simulink model "Planta_Matlab"  (R2017a)
settings: Solver=VariableStepAuto  StartTime=0.0  StopTime=0.4  MaxStep=1e-4  RelTol=1e-3
libraries: powerlib x20, opclib x10, simulink x7, powerlib_meascontrol x3, re_lib x1
settings Model: Creator=lideq2  LastModifiedBy=igor-
settings SolverCC: MaxConsecutiveZCs=10000

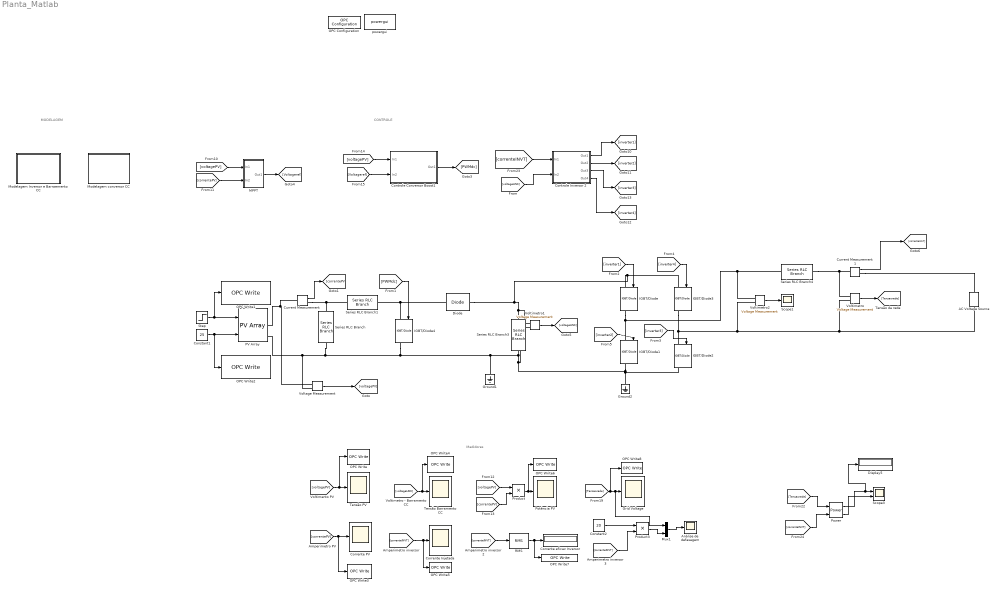
== system Planta_Matlab ==
  note: CONTROLE
  note: Medidores
  note: MODELAGEM
  AC Voltage Source : powerlib/Electrical Sources/AC Voltage Source  Amplitude=325  Phase=0  Frequency=60  SampleTime=0  Measurements=None  BusType=swing  Pref=10e3  Qref=0  Qmin=-inf  Qmax=+inf
  Análise de defasagem : Scope
  Constant1 : Constant  Value=25
  Constant2 : Constant  Value=20
  Controle Conversor Boost1 : Subsystem
  Controle Inversor 2 : Subsystem
  Corrente Injetada : Scope
  "Corrente PV " : Scope
  Corrente eficaz Inversor : Display
  Current Measurement : powerlib/Measurements/Current Measurement  PhasorSimulation=off  OutputType=Complex  PSBequivalent=0
  Current Measurement1 : powerlib/Measurements/Current Measurement  PhasorSimulation=off  OutputType=Complex  PSBequivalent=0
  Diode : powerlib/Power Electronics/Diode  Ron=0.001  Lon=0  Vf=0.8  IC=0  UseSnubber=off  Rs=500  Cs=250e-9  Measurements=off
  Display5 : Display
  Grid Voltage : Scope
  Ground1 : powerlib/Elements/Ground  LConnTagsString=a
  Ground2 : powerlib/Elements/Ground  LConnTagsString=a
  IGBT/Diode{,1..4} (5 alike) : powerlib/Power Electronics/IGBT//Diode  Ron=1e-3  Rs=1e5  Cs=inf  Measurements=on
  MPPT : Subsystem
  Modelagem Inversor e Barraemento CC : Subsystem
  Modelagem conversor CC : Subsystem
  Mux1 : Mux  Inputs=2
  OPC Configuration : opclib/OPC Configuration  opcServers=localhost/Matrikon.OPC.Simulation.1/10  errMissingItems=Error  errReadWrite=Warn  errShutdown=Error  errRTViolation=Warn  rtEnable=on  speedup=1  showLatency=off  beingUsed=on
      settings: SourceProductName=OPC Toolbox  SourceProductBaseCode=OT
  OPC Write : opclib/OPC Write  serverHost=localhost  serverID=Matrikon.OPC.Simulation.1  itemIDs=PV_v2.Placa.Tensão_PV  writeMode=Synchronous  updateRate=0
      settings: SourceProductName=OPC Toolbox  SourceProductBaseCode=OT
  OPC Write1 : opclib/OPC Write  serverHost=localhost  serverID=Matrikon.OPC.Simulation.1  itemIDs=PV_v2.Placa.IRRADIANCIA  writeMode=Synchronous  updateRate=0
      settings: SourceProductName=OPC Toolbox  SourceProductBaseCode=OT
  OPC Write2 : opclib/OPC Write  serverHost=localhost  serverID=Matrikon.OPC.Simulation.1  itemIDs=PV_v2.Placa.TEMPERATURA  writeMode=Synchronous  updateRate=0
      settings: SourceProductName=OPC Toolbox  SourceProductBaseCode=OT
  OPC Write3 : opclib/OPC Write  serverHost=localhost  serverID=Matrikon.OPC.Simulation.1  itemIDs=PV_v2.Placa.Corrente_PV  writeMode=Synchronous  updateRate=0
      settings: SourceProductName=OPC Toolbox  SourceProductBaseCode=OT
  OPC Write4 : opclib/OPC Write  serverHost=localhost  serverID=Matrikon.OPC.Simulation.1  itemIDs=PV_v2.Placa.Tensão_Barramento  writeMode=Synchronous  updateRate=0
      settings: SourceProductName=OPC Toolbox  SourceProductBaseCode=OT
  OPC Write5 : opclib/OPC Write  serverHost=localhost  serverID=Matrikon.OPC.Simulation.1  itemIDs=PV_v2.Inversor.Corrente_Injetada  writeMode=Synchronous  updateRate=0
      settings: SourceProductName=OPC Toolbox  SourceProductBaseCode=OT
  OPC Write6 : opclib/OPC Write  serverHost=localhost  serverID=Matrikon.OPC.Simulation.1  itemIDs=PV_v2.Placa.Potência_PV  writeMode=Synchronous  updateRate=0
      settings: SourceProductName=OPC Toolbox  SourceProductBaseCode=OT
  OPC Write7 : opclib/OPC Write  serverHost=localhost  serverID=Matrikon.OPC.Simulation.1  itemIDs=PV_v2.Inversor.Corrente_Eficaz_INV  writeMode=Synchronous  updateRate=0
      settings: SourceProductName=OPC Toolbox  SourceProductBaseCode=OT
  OPC Write8 : opclib/OPC Write  serverHost=localhost  serverID=Matrikon.OPC.Simulation.1  itemIDs=PV_v2.Rede.Tensão_Rede  writeMode=Synchronous  updateRate=0
      settings: SourceProductName=OPC Toolbox  SourceProductBaseCode=OT
  PV Array : re_lib/Solar/PV Array  Npar=1  Nser=5  PlotType=array @ 1000 W/m2 & specified temperatures  S_vec="[ 1000  500  100 ]"  Temp_C_vec="[ 45 25  ]"  ModuleName=Yingli Energy (China) YL240P-29b  PlotWhenSelected=off  Pm=240.13  Ncell=60  Voc=37.5  Isc=8.65  Vm=29.5  Im=8.14  beta_Voc_pc=-0.33701  alpha_Isc_pc=0.043803  beta_Voc=-0.12638  alpha_Isc=0.003789  IL=8.6929  I0=1.2567e-10  nI=0.97513  Rsh=337.0126  Rs=0.44582  BAL=off  Tc=1e-6  Tfilter=5e-5
  Potência PV : Scope
  Power : powerlib_meascontrol/Measurements/Power  Freq=60  Vinit=[1, 0]  Iinit=[1, 0]  Ts=1e-6
      settings: SourceProductName=Simscape Power Systems
  Product : Product
  Product3 : Product
  RMS : powerlib_meascontrol/Measurements/RMS  TrueRMS=on  Freq=60  RMSInit=120  Ts=0
  Scope1 : Scope
  Scope3 : Scope  NumInputPorts=2
  Series RLC Branch : powerlib/Elements/Series RLC Branch  LConnTagsString=__new0  RConnTagsString=__new0  BranchType=C  Resistance=1  Inductance=1e-3  SetiL0=off  InitialCurrent=0  Capacitance=1e-3  Setx0=off  InitialVoltage=0  Measurements=None
  Series RLC Branch1 : powerlib/Elements/Series RLC Branch  LConnTagsString=__new0  RConnTagsString=__new0  BranchType=L  Resistance=1  Inductance=71*10^-3  SetiL0=off  InitialCurrent=0  Capacitance=1e-6  Setx0=off  InitialVoltage=0  Measurements=None
  Series RLC Branch3 : powerlib/Elements/Series RLC Branch  LConnTagsString=__new0  RConnTagsString=__new0  BranchType=C  Resistance=1  Inductance=1e-3  SetiL0=off  InitialCurrent=0  Capacitance=1e-3  Setx0=off  InitialVoltage=400  Measurements=None
  Series RLC Branch4 : powerlib/Elements/Series RLC Branch  LConnTagsString=__new0  RConnTagsString=__new0  BranchType=RL  Resistance=0.05  Inductance=2.2e-3  SetiL0=off  InitialCurrent=0  Capacitance=1e-6  Setx0=off  InitialVoltage=0  Measurements=None
  Step : Step  Time=0.2  Before=1000  After=500  SampleTime=0
  Tensão Barramento CC : Scope
  Tensão PV : Scope
  Voltage Measurement : powerlib/Measurements/Voltage Measurement  PhasorSimulation=off  OutputType=Complex  PSBequivalent=0
  Voltimetro : powerlib/Measurements/Voltage Measurement  PhasorSimulation=off  OutputType=Complex  PSBequivalent=0
  Voltimetro1 : powerlib/Measurements/Voltage Measurement  PhasorSimulation=off  OutputType=Complex  PSBequivalent=0
  Voltimetro2 : powerlib/Measurements/Voltage Measurement  PhasorSimulation=off  OutputType=Complex  PSBequivalent=0
  powergui : powerlib/powergui  Priority=1  SimulationMode=Continuous  SampleTime=1e-6  frequency=60  Iterations=50  frequencyindice=0  Pbase=100e6  ErrMax=1e-4  UnitsV=kV  UnitsW=MW  buscounter=0  FunctionMessages=off  echomessages=off  EnableUseOfTLC=off  CurrentSourceSwitches=off  DisableSnubberDevices=off  DisableRonSwitches=off  DisableVfSwitches=off  DisplayEquations=off  SolverType=Tustin/Backward Euler (TBE)  Interpol=off  ExternalGateDelay=off  methode=off  Ts=100  x0status=blocks  SPID=on  SwTol=0  HookPort=off  RestoreLinks=warning  ResistiveCurrentMeasurement=off  Frange=[0:2:500]  Ylog=off  Xlog=on  ShowGrid=off  save=off  variable=ZData  structure=0  ZoomFFT=off  StartTime=0.0  cycles=1  DisplayStyle=1  fundamental=60  FreqAxis=off  MaxFrequency=1000  frequencyindicesteady=1  RmsSteady=1  display=off
  wires:
  Constant1/1 -> OPC Write2/1, PV Array/2
  Step/1 -> OPC Write1/1, PV Array/1
  Voltage Measurement/1 -> [voltagePV]
  Current Measurement/1 -> [correntePV]
  [inverter1] -> IGBT/Diode/1
  [inverter3] -> IGBT/Diode2/1
  [inverter4] -> IGBT/Diode3/1
  [inverter2] -> IGBT/Diode1/1
  [voltagePV] -> OPC Write/1, Tensão PV/1
  [correntePV] -> "Corrente PV "/1, OPC Write3/1
  Current Measurement1/1 -> [correnteINVT]
  [voltageLINK] -> OPC Write4/1, Tensão Barramento CC/1
  [correnteINVT] -> OPC Write5/1, Corrente Injetada/1
  [voltagePV] -> Controle Conversor Boost1/1(In1)
  Controle Conversor Boost1/1(Out1) -> [PWMdc]
  [Voltageref] -> Controle Conversor Boost1/2(In2)
  [voltagePV] -> MPPT/1(In1)
  [correntePV] -> MPPT/2(In2)
  MPPT/1(Out1) -> [Voltageref]
  Product/1 -> OPC Write6/1, Potência PV/1
  [voltagePV] -> Product/1
  [correntePV] -> Product/2
  Voltimetro/1 -> [Tensaorede]
  [Tensaorede] -> Mux1/1, Grid Voltage/1, OPC Write8/1
  [PWMdc] -> IGBT/Diode4/1
  Voltimetro1/1 -> [voltageLINK]
  Voltimetro2/1 -> Scope1/1
  RMS/1 -> OPC Write7/1, Corrente eficaz Inversor/1
  [correnteINVT] -> RMS/1
  [correnteINVT] -> Controle Inversor 2/1(In1)
  Controle Inversor 2/1(Out1) -> [inverter1]
  Controle Inversor 2/2(Out2) -> [inverter2]
  Controle Inversor 2/4(Out4) -> [inverter4]
  Controle Inversor 2/3(Out3) -> [inverter3]
  [voltageLINK] -> Controle Inversor 2/2(In2)
  [Tensaorede] -> Power/1
  [correnteINVT] -> Power/2
  Power/1 -> Display5/1, Scope3/1
  Power/2 -> Scope3/2
  [correnteINVT] -> Product3/2
  Constant2/1 -> Product3/1
  Product3/1 -> Mux1/2
  Mux1/1 -> Análise de defasagem/1
  connections:
  Series RLC Branch/RConn1 -- Voltimetro1/LConn2 -- Ground2/LConn1 -- IGBT/Diode2/RConn1 -- IGBT/Diode1/RConn1 -- Series RLC Branch3/RConn1 -- Ground1/LConn1 -- IGBT/Diode4/RConn1 -- Voltage Measurement/LConn2 -- PV Array/RConn2
  Voltage Measurement/LConn1 -- Current Measurement/LConn1 -- PV Array/RConn1
  Diode/LConn1 -- Series RLC Branch1/RConn1 -- IGBT/Diode4/LConn1
  Series RLC Branch/LConn1 -- Current Measurement/RConn1 -- Series RLC Branch1/LConn1
  IGBT/Diode/RConn1 -- Series RLC Branch4/LConn1 -- Voltimetro2/LConn1 -- IGBT/Diode1/LConn1
  IGBT/Diode3/RConn1 -- Voltimetro2/LConn2 -- Voltimetro/LConn2 -- AC Voltage Source/LConn1 -- IGBT/Diode2/LConn1
  Current Measurement1/RConn1 -- AC Voltage Source/RConn1
  Series RLC Branch4/RConn1 -- Voltimetro/LConn1 -- Current Measurement1/LConn1
  IGBT/Diode3/LConn1 -- Voltimetro1/LConn1 -- Series RLC Branch3/LConn1 -- Diode/RConn1 -- IGBT/Diode/LConn1

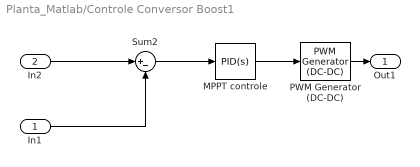
== system Planta_Matlab/Controle Conversor Boost1 ==
  In1 : Inport
  In2 : Inport  Port=2
  MPPT controle : simulink/Continuous/PID Controller  Controller=PID  TimeDomain=Continuous-time  SampleTime=-1  IntegratorMethod=Forward Euler  FilterMethod=Forward Euler  Form=Parallel  UseFilter=on  ControllerParametersSource=internal  P=-0.096886640335999  I=-17.7155282909639  D=-0.000128015040144556  N=10858.1536805525  InitialConditionSource=internal  InitialConditionForIntegrator=0  InitialConditionForFilter=0  ExternalReset=none  LimitOutput=off  UpperSaturationLimit=inf  LowerSaturationLimit=-inf  LinearizeAsGain=on  AntiWindupMode=none  Kb=1  TrackingMode=off  Kt=1  PParamMin=[]  PParamMax=[]  IParamMin=[]  IParamMax=[]  DParamMin=[]  DParamMax=[]  NParamMin=[]  NParamMax=[]  KbParamMin=[]  KbParamMax=[]  KtParamMin=[]  KtParamMax=[]  POutMin=[]  POutMax=[]  IOutMin=[]  IOutMax=[]  DOutMin=[]  DOutMax=[]  NOutMin=[]  NOutMax=[]  KbOutMin=[]  KbOutMax=[]  KtOutMin=[]  KtOutMax=[]  IntegratorOutMin=[]  IntegratorOutMax=[]  FilterOutMin=[]  FilterOutMax=[]  SumOutMin=[]  SumOutMax=[]  SumI1OutMin=[]  SumI1OutMax=[]  SumI2OutMin=[]  SumI2OutMax=[]  SumI3OutMin=[]  SumI3OutMax=[]  SumDOutMin=[]  SumDOutMax=[]  SaturationOutMin=[]  SaturationOutMax=[]  IntegratorContinuousStateAttributes=''  IntegratorStateMustResolveToSignalObject=off  IntegratorRTWStateStorageClass=Auto  FilterContinuousStateAttributes=''  FilterStateMustResolveToSignalObject=off  FilterRTWStateStorageClass=Auto  DifferentiatorICPrevScaledInput=0  DifferentiatorOutMin=[]  DifferentiatorOutMax=[]  InitialConditionSetting=State (most efficient)
  PWM Generator (DC-DC) : powerlib_meascontrol/Pulse & Signal Generators/PWM Generator (DC-DC)  Fsw=10000  Ts=0
  Sum2 : Sum  Inputs=|+-
  Out1 : Outport
  wires:
  In2/1 -> Sum2/1
  Sum2/1 -> MPPT controle/1
  MPPT controle/1 -> PWM Generator (DC-DC)/1
  In1/1 -> Sum2/2
  PWM Generator (DC-DC)/1 -> Out1/1

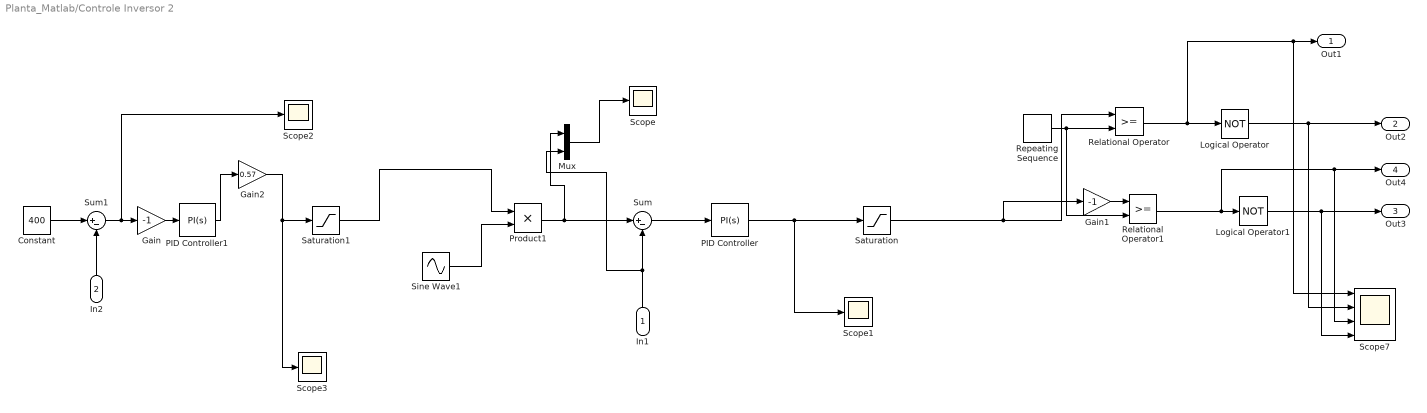
== system Planta_Matlab/Controle Inversor 2 ==
  In1 : Inport
  In2 : Inport  Port=2
  Constant : Constant  Value=400
  Gain : Gain  Gain=-1
  Gain1 : Gain  Gain=-1
  Gain2 : Gain  Gain=0.57
  Logical Operator : Logic  Operator=NOT  AllPortsSameDT=off  OutDataTypeStr=boolean
  Logical Operator1 : Logic  Operator=NOT  AllPortsSameDT=off  OutDataTypeStr=boolean
  Mux : Mux  Inputs=2
  PID Controller : simulink/Continuous/PID Controller  Controller=PI  TimeDomain=Continuous-time  SampleTime=-1  IntegratorMethod=Forward Euler  FilterMethod=Forward Euler  Form=Parallel  UseFilter=on  ControllerParametersSource=internal  P=10  I=0.00001  D=0  N=100  InitialConditionSource=internal  InitialConditionForIntegrator=0  InitialConditionForFilter=0  ExternalReset=none  LimitOutput=off  UpperSaturationLimit=inf  LowerSaturationLimit=-inf  LinearizeAsGain=on  AntiWindupMode=none  Kb=1  TrackingMode=off  Kt=1  PParamMin=[]  PParamMax=[]  IParamMin=[]  IParamMax=[]  DParamMin=[]  DParamMax=[]  NParamMin=[]  NParamMax=[]  KbParamMin=[]  KbParamMax=[]  KtParamMin=[]  KtParamMax=[]  POutMin=[]  POutMax=[]  IOutMin=[]  IOutMax=[]  DOutMin=[]  DOutMax=[]  NOutMin=[]  NOutMax=[]  KbOutMin=[]  KbOutMax=[]  KtOutMin=[]  KtOutMax=[]  IntegratorOutMin=[]  IntegratorOutMax=[]  FilterOutMin=[]  FilterOutMax=[]  SumOutMin=[]  SumOutMax=[]  SumI1OutMin=[]  SumI1OutMax=[]  SumI2OutMin=[]  SumI2OutMax=[]  SumI3OutMin=[]  SumI3OutMax=[]  SumDOutMin=[]  SumDOutMax=[]  SaturationOutMin=[]  SaturationOutMax=[]  IntegratorContinuousStateAttributes=''  IntegratorStateMustResolveToSignalObject=off  IntegratorRTWStateStorageClass=Auto  FilterContinuousStateAttributes=''  FilterStateMustResolveToSignalObject=off  FilterRTWStateStorageClass=Auto  DifferentiatorICPrevScaledInput=0  DifferentiatorOutMin=[]  DifferentiatorOutMax=[]  InitialConditionSetting=State (most efficient)
  PID Controller1 : simulink/Continuous/PID Controller  Controller=PI  TimeDomain=Continuous-time  SampleTime=-1  IntegratorMethod=Forward Euler  FilterMethod=Forward Euler  Form=Parallel  UseFilter=on  ControllerParametersSource=internal  P=0.5  I=50  D=0  N=100  InitialConditionSource=internal  InitialConditionForIntegrator=0  InitialConditionForFilter=0  ExternalReset=none  LimitOutput=off  UpperSaturationLimit=inf  LowerSaturationLimit=-inf  LinearizeAsGain=on  AntiWindupMode=none  Kb=1  TrackingMode=off  Kt=1  PParamMin=[]  PParamMax=[]  IParamMin=[]  IParamMax=[]  DParamMin=[]  DParamMax=[]  NParamMin=[]  NParamMax=[]  KbParamMin=[]  KbParamMax=[]  KtParamMin=[]  KtParamMax=[]  POutMin=[]  POutMax=[]  IOutMin=[]  IOutMax=[]  DOutMin=[]  DOutMax=[]  NOutMin=[]  NOutMax=[]  KbOutMin=[]  KbOutMax=[]  KtOutMin=[]  KtOutMax=[]  IntegratorOutMin=[]  IntegratorOutMax=[]  FilterOutMin=[]  FilterOutMax=[]  SumOutMin=[]  SumOutMax=[]  SumI1OutMin=[]  SumI1OutMax=[]  SumI2OutMin=[]  SumI2OutMax=[]  SumI3OutMin=[]  SumI3OutMax=[]  SumDOutMin=[]  SumDOutMax=[]  SaturationOutMin=[]  SaturationOutMax=[]  IntegratorContinuousStateAttributes=''  IntegratorStateMustResolveToSignalObject=off  IntegratorRTWStateStorageClass=Auto  FilterContinuousStateAttributes=''  FilterStateMustResolveToSignalObject=off  FilterRTWStateStorageClass=Auto  DifferentiatorICPrevScaledInput=0  DifferentiatorOutMin=[]  DifferentiatorOutMax=[]  InitialConditionSetting=State (most efficient)
  Product1 : Product
  Relational Operator : RelationalOperator  OutDataTypeStr=boolean  ZeroCross=off  RndMeth=Simplest
  Relational Operator1 : RelationalOperator  OutDataTypeStr=boolean  ZeroCross=off  RndMeth=Simplest
  Repeating Sequence : simulink/Sources/Repeating Sequence  rep_seq_t=[0 1 2]*(1/20000)  rep_seq_y=[1 -1 1]
  Saturation : Saturate  UpperLimit=1  LowerLimit=-1
  Saturation1 : Saturate  UpperLimit=15  LowerLimit=-15
  Scope{,1..3} (4 alike) : Scope
  Scope7 : Scope  NumInputPorts=4
  Sine Wave1 : Sin  Frequency=2*pi*60  SampleTime=0
  Sum : Sum  Inputs=|+-
  Sum1 : Sum  Inputs=|+-
  Out1 : Outport
  Out2 : Outport  Port=2
  Out3 : Outport  Port=3
  Out4 : Outport  Port=4
  wires:
  Relational Operator1/1 -> Scope7/3, Out4/1, Logical Operator1/1
  Logical Operator1/1 -> Out3/1, Scope7/4
  Relational Operator/1 -> Scope7/1, Out1/1, Logical Operator/1
  Logical Operator/1 -> Scope7/2, Out2/1
  Repeating Sequence/1 -> Relational Operator1/2, Relational Operator/2
  Gain1/1 -> Relational Operator1/1
  PID Controller1/1 -> Gain2/1
  Sine Wave1/1 -> Product1/2
  Product1/1 -> Mux/1, Sum/1
  In1/1 -> Mux/2, Sum/2
  Sum/1 -> PID Controller/1
  PID Controller/1 -> Scope1/1, Saturation/1
  Mux/1 -> Scope/1
  Saturation/1 -> Gain1/1, Relational Operator/1
  In2/1 -> Sum1/2
  Constant/1 -> Sum1/1
  Sum1/1 -> Scope2/1, Gain/1
  Saturation1/1 -> Product1/1
  Gain/1 -> PID Controller1/1
  Gain2/1 -> Scope3/1, Saturation1/1

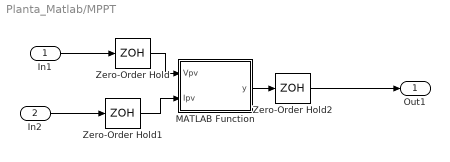
== system Planta_Matlab/MPPT ==
  In1 : Inport
  In2 : Inport  Port=2
  MATLAB Function : MATLAB Function  TreatAsAtomicUnit=on
  Zero-Order Hold : ZeroOrderHold  SampleTime=-1
  Zero-Order Hold1 : ZeroOrderHold  SampleTime=-1
  Zero-Order Hold2 : ZeroOrderHold  SampleTime=-1
  Out1 : Outport
  wires:
  In1/1 -> Zero-Order Hold/1
  Zero-Order Hold1/1 -> MATLAB Function/2(Ipv)
  In2/1 -> Zero-Order Hold1/1
  Zero-Order Hold/1 -> MATLAB Function/1(Vpv)
  Zero-Order Hold2/1 -> Out1/1
  MATLAB Function/1(y) -> Zero-Order Hold2/1

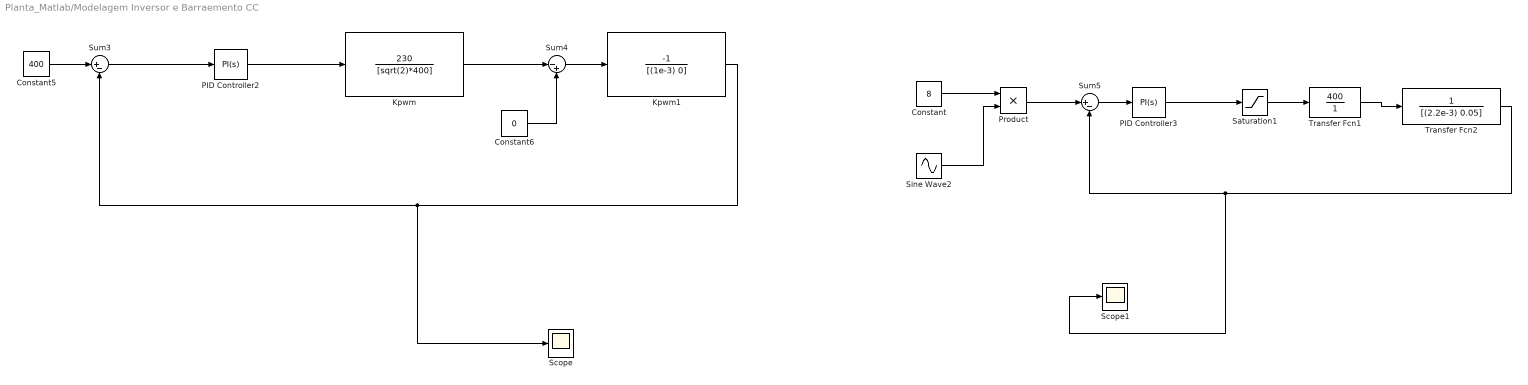
== system Planta_Matlab/Modelagem Inversor e Barraemento CC ==
  Constant : Constant  Value=8
  Constant5 : Constant  Value=400
  Constant6 : Constant  Value=0
  Kpwm : TransferFcn  Numerator=[ 230]  Denominator=[sqrt(2)*400]
  Kpwm1 : TransferFcn  Numerator=[-1]  Denominator=[(1e-3) 0]
  PID Controller2 : simulink/Continuous/PID Controller  Controller=PI  TimeDomain=Continuous-time  SampleTime=-1  IntegratorMethod=Forward Euler  FilterMethod=Forward Euler  Form=Parallel  UseFilter=on  ControllerParametersSource=internal  P=0.00212999108068102  I=0.00122975092380269  D=0  N=100  InitialConditionSource=internal  InitialConditionForIntegrator=0  InitialConditionForFilter=0  ExternalReset=none  LimitOutput=off  UpperSaturationLimit=inf  LowerSaturationLimit=-inf  LinearizeAsGain=on  AntiWindupMode=none  Kb=1  TrackingMode=off  Kt=1  PParamMin=[]  PParamMax=[]  IParamMin=[]  IParamMax=[]  DParamMin=[]  DParamMax=[]  NParamMin=[]  NParamMax=[]  KbParamMin=[]  KbParamMax=[]  KtParamMin=[]  KtParamMax=[]  POutMin=[]  POutMax=[]  IOutMin=[]  IOutMax=[]  DOutMin=[]  DOutMax=[]  NOutMin=[]  NOutMax=[]  KbOutMin=[]  KbOutMax=[]  KtOutMin=[]  KtOutMax=[]  IntegratorOutMin=[]  IntegratorOutMax=[]  FilterOutMin=[]  FilterOutMax=[]  SumOutMin=[]  SumOutMax=[]  SumI1OutMin=[]  SumI1OutMax=[]  SumI2OutMin=[]  SumI2OutMax=[]  SumI3OutMin=[]  SumI3OutMax=[]  SumDOutMin=[]  SumDOutMax=[]  SaturationOutMin=[]  SaturationOutMax=[]  IntegratorContinuousStateAttributes=''  IntegratorStateMustResolveToSignalObject=off  IntegratorRTWStateStorageClass=Auto  FilterContinuousStateAttributes=''  FilterStateMustResolveToSignalObject=off  FilterRTWStateStorageClass=Auto  DifferentiatorICPrevScaledInput=0  DifferentiatorOutMin=[]  DifferentiatorOutMax=[]  InitialConditionSetting=State (most efficient)
  PID Controller3 : simulink/Continuous/PID Controller  Controller=PI  TimeDomain=Continuous-time  SampleTime=-1  IntegratorMethod=Forward Euler  FilterMethod=Forward Euler  Form=Parallel  UseFilter=on  ControllerParametersSource=internal  P=10  I=0.00001  D=0  N=100  InitialConditionSource=internal  InitialConditionForIntegrator=0  InitialConditionForFilter=0  ExternalReset=none  LimitOutput=off  UpperSaturationLimit=inf  LowerSaturationLimit=-inf  LinearizeAsGain=on  AntiWindupMode=none  Kb=1  TrackingMode=off  Kt=1  PParamMin=[]  PParamMax=[]  IParamMin=[]  IParamMax=[]  DParamMin=[]  DParamMax=[]  NParamMin=[]  NParamMax=[]  KbParamMin=[]  KbParamMax=[]  KtParamMin=[]  KtParamMax=[]  POutMin=[]  POutMax=[]  IOutMin=[]  IOutMax=[]  DOutMin=[]  DOutMax=[]  NOutMin=[]  NOutMax=[]  KbOutMin=[]  KbOutMax=[]  KtOutMin=[]  KtOutMax=[]  IntegratorOutMin=[]  IntegratorOutMax=[]  FilterOutMin=[]  FilterOutMax=[]  SumOutMin=[]  SumOutMax=[]  SumI1OutMin=[]  SumI1OutMax=[]  SumI2OutMin=[]  SumI2OutMax=[]  SumI3OutMin=[]  SumI3OutMax=[]  SumDOutMin=[]  SumDOutMax=[]  SaturationOutMin=[]  SaturationOutMax=[]  IntegratorContinuousStateAttributes=''  IntegratorStateMustResolveToSignalObject=off  IntegratorRTWStateStorageClass=Auto  FilterContinuousStateAttributes=''  FilterStateMustResolveToSignalObject=off  FilterRTWStateStorageClass=Auto  DifferentiatorICPrevScaledInput=0  DifferentiatorOutMin=[]  DifferentiatorOutMax=[]  InitialConditionSetting=State (most efficient)
  Product : Product
  Saturation1 : Saturate  UpperLimit=0.8  LowerLimit=0
  Scope : Scope
  Scope1 : Scope
  Sine Wave2 : Sin  Frequency=2*pi*60  SampleTime=0
  Sum3 : Sum  Inputs=|+-
  Sum4 : Sum  Inputs=|-+
  Sum5 : Sum  Inputs=|+-
  Transfer Fcn1 : TransferFcn  Numerator=[400]  Denominator=[1]
  Transfer Fcn2 : TransferFcn  Denominator=[(2.2e-3) 0.05]
  wires:
  Kpwm1/1 -> Scope/1, Sum3/2
  Constant5/1 -> Sum3/1
  Sum3/1 -> PID Controller2/1
  Constant6/1 -> Sum4/2
  PID Controller2/1 -> Kpwm/1
  PID Controller3/1 -> Saturation1/1
  Transfer Fcn1/1 -> Transfer Fcn2/1
  Sum5/1 -> PID Controller3/1
  Saturation1/1 -> Transfer Fcn1/1
  Sum4/1 -> Kpwm1/1
  Product/1 -> Sum5/1
  Kpwm/1 -> Sum4/1
  Sine Wave2/1 -> Product/2
  Constant/1 -> Product/1
  Transfer Fcn2/1 -> Scope1/1, Sum5/2

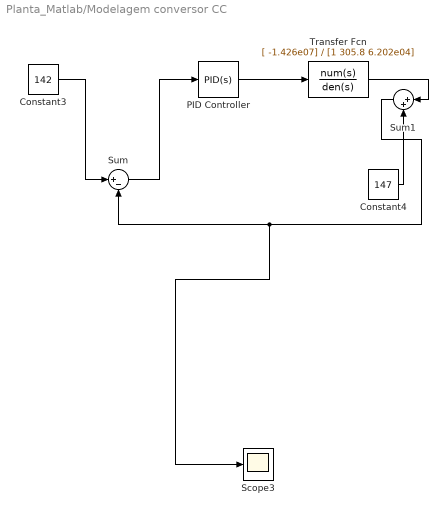
== system Planta_Matlab/Modelagem conversor CC ==
  Constant3 : Constant  Value=142
  Constant4 : Constant  Value=147
  PID Controller : simulink/Continuous/PID Controller  Controller=PID  TimeDomain=Continuous-time  SampleTime=-1  IntegratorMethod=Forward Euler  FilterMethod=Forward Euler  Form=Parallel  UseFilter=on  ControllerParametersSource=internal  P=-0.096886640335999  I=-17.7155282909639  D=-0.000128015040144556  N=10858.1536805525  InitialConditionSource=internal  InitialConditionForIntegrator=0  InitialConditionForFilter=0  ExternalReset=none  LimitOutput=off  UpperSaturationLimit=inf  LowerSaturationLimit=-inf  LinearizeAsGain=on  AntiWindupMode=none  Kb=1  TrackingMode=off  Kt=1  PParamMin=[]  PParamMax=[]  IParamMin=[]  IParamMax=[]  DParamMin=[]  DParamMax=[]  NParamMin=[]  NParamMax=[]  KbParamMin=[]  KbParamMax=[]  KtParamMin=[]  KtParamMax=[]  POutMin=[]  POutMax=[]  IOutMin=[]  IOutMax=[]  DOutMin=[]  DOutMax=[]  NOutMin=[]  NOutMax=[]  KbOutMin=[]  KbOutMax=[]  KtOutMin=[]  KtOutMax=[]  IntegratorOutMin=[]  IntegratorOutMax=[]  FilterOutMin=[]  FilterOutMax=[]  SumOutMin=[]  SumOutMax=[]  SumI1OutMin=[]  SumI1OutMax=[]  SumI2OutMin=[]  SumI2OutMax=[]  SumI3OutMin=[]  SumI3OutMax=[]  SumDOutMin=[]  SumDOutMax=[]  SaturationOutMin=[]  SaturationOutMax=[]  IntegratorContinuousStateAttributes=''  IntegratorStateMustResolveToSignalObject=off  IntegratorRTWStateStorageClass=Auto  FilterContinuousStateAttributes=''  FilterStateMustResolveToSignalObject=off  FilterRTWStateStorageClass=Auto  DifferentiatorICPrevScaledInput=0  DifferentiatorOutMin=[]  DifferentiatorOutMax=[]  InitialConditionSetting=State (most efficient)
  Scope3 : Scope
  Sum : Sum  Inputs=|+-
  Sum1 : Sum  Inputs=|++
  Transfer Fcn : TransferFcn  Numerator=[ -1.426e07]  Denominator=[1 305.8 6.202e04]
  wires:
  PID Controller/1 -> Transfer Fcn/1
  Constant3/1 -> Sum/1
  Sum1/1 -> Scope3/1, Sum/2
  Constant4/1 -> Sum1/2
  Sum/1 -> PID Controller/1
  Transfer Fcn/1 -> Sum1/1

== matlab function Planta_Matlab/MPPT/MATLAB Function ==
  data: Vpv input; y output; Ipv input
function y = fcn(Vpv,Ipv)
%Define internal values fot the voltage and power as persistent
persistent Pprev Vprev

% Initialize the internal Values for the voltage and power on the first
% pass

if isempty(Vprev)
    Vprev = 147.5;
    Pprev = 1201;
end

% Initialize algorithm paramaters
deltaD = 0.0001;

% Calculate measured array power
Ppv = Vpv*Ipv;

% Increase or decrease duty cycle based on conditions
if (Ppv - Pprev) ~= 0 
    if(Ppv-Pprev) > 0 
        if(Vpv-Vprev) > 0
            Vref = Vprev + deltaD;
        else
            Vref = Vprev - deltaD;
        end
    else
        if(Vpv-Vprev) > 0
            Vref = Vprev - deltaD;
        else
            Vref = Vprev + deltaD;
        end
    end
else
    Vref = Vprev;
end

%Update internal values
Vprev = Vref;
Pprev = Ppv;

y = Vref;
